simulink model "simTopLevel"  (R2016b)
settings: Solver=ode15s  StartTime=0.0  StopTime=2  RelTol=1e-3  EnableMultiTasking=on
InitFcn:
  | % minitaurParameters
model workspace (MAT data in the model file):
  MCOS : class17 (value not decoded)
  MCOS : class17 (value not decoded)
  MCOS : class17 (value not decoded)
  MCOS : class17 (value not decoded)
values from neighbouring files (symbols this model uses):
  controlParams = Simulink.Parameter(controlParams)    [minitaurParameters.m]
  envParams = Simulink.Parameter(envParams)    [minitaurParameters.m]
  IC = Simulink.Parameter(IC)    [minitaurParameters.m]
  minitaurParams = Simulink.Parameter(minitaurParams)    [minitaurParameters.m]
undefined symbols (not defined in the file or in its folder): Axis, Fn, ForeRearLag, Period, tau0, tau1, X, Y, Z
libraries: sm_lib x464, fl_lib x132, nesl_utility x41, Contact_Forces_Lib x28, simulink x13, simulink_extras x1
(part 13 of 13)

== system simTopLevel/GR Minitaur/minitaur_motor_module_IVB/DYS_BLDC_86x10_BE8108_12/DYS_BLDC_86x10_BE8108_12_stator_1_RIGID ==
  ReferenceFrame : sm_lib/Frames and Transforms/Reference Frame
  Solid : sm_lib/Body Elements/Solid  InertiaType=Custom  Mass=minitaurParams.Solid(6).mass  MassUnits=kg  CenterOfMass=minitaurParams.Solid(6).CoM  CenterOfMassUnits=mm  MomentsOfInertia=minitaurParams.Solid(6).MoI  MomentsOfInertiaUnits=kg*mm^2  ProductsOfInertia=minitaurParams.Solid(6).PoI  ProductsOfInertiaUnits=kg*mm^2  DensityBased=on  Density=1000  DensityUnits=kg/(m^3)  DoExposeReferenceFrame=on  SerializedFrames=<Frames/>  GraphicType=FromGeometry  MarkerShape=Sphere  MarkerSize=10  GraphicVisPropType=SimpleVisualProperties  GraphicDiffuseColor=minitaurParams.Solid(6).color  GraphicSpecularColor=[0.5 0.5 0.5 1.0]  GraphicAmbientColor=[0.15 0.15 0.15 1.0]  GraphicEmissiveColor=[0.0 0.0 0.0 1.0]  GraphicShininess=75  GraphicOpacity=minitaurParams.Solid(6).opacity  GeometryShape=FromFile  RectangleSize=[1 1]  RectangleSizeUnits=m  BrickDimensions=[1 1 1]  BrickDimensionUnits=m  CylinderRadius=1  CylinderRadiusUnits=m  CylinderLength=1  CylinderLengthUnits=m  SphereRadius=1  SphereRadiusUnits=m  EllipsoidRadii=[1 1 1]  EllipsoidRadiiUnits=m  ExtrusionCrossSection=[1 1; -1 1; -1 -1; 1 -1]  ExtrusionCrossSectionUnits=m  ExtrusionLength=1  ExtrusionLengthUnits=m  PolygonNumSides=3  PolygonOuterRadius=1  PolygonOuterRadiusUnits=m  ExtGeomFileType=STEP  ExtGeomFileName=model/DYS-BLDC-86x10-BE8108-12-stator_Default_sldprt.STEP  ExtGeomFileUnits=m  RevolutionCrossSection=[1 1; 1 -1; 2 -1; 2 1]  RevolutionCrossSectionUnits=m  RevolutionExtent=Full  RevolutionAngle=180  RevolutionAngleUnits=deg
  Transform : sm_lib/Frames and Transforms/Rigid Transform  TranslationMethod=Cartesian  TranslationStandardOffset=0  TranslationLengthUnit=mm  TranslationStandardAxis=+Z  TranslationCartesianOffset=minitaurParams.RigidTransform(17).translation  TranslationROffset=0  TranslationROffsetUnits=m  TranslationZOffset=0  TranslationZOffsetUnits=m  TranslationThetaOffset=0  TranslationThetaOffsetUnits=deg  RotationMethod=ArbitraryAxis  RotationAngleUnits=rad  RotationStandardAxis=+Z  RotationAngle=minitaurParams.RigidTransform(17).angle  RotationArbitraryAxis=minitaurParams.RigidTransform(17).axis  FollAlignAxisA=+X  BaseAlignAxisA=+Y  FollAlignAxisB=+Y  BaseAlignAxisB=+Z  RotationSequenceAxes=FollowerAxes  RotationSequence=XYX  RotationSequenceAngles=[0 0 0]  RotationSequenceAnglesUnits=deg  RotationMatrix=[1 0 0; 0 1 0; 0 0 1]
  Transform1 : sm_lib/Frames and Transforms/Rigid Transform  TranslationMethod=Cartesian  TranslationStandardOffset=0  TranslationLengthUnit=mm  TranslationStandardAxis=+Z  TranslationCartesianOffset=minitaurParams.RigidTransform(19).translation  TranslationROffset=0  TranslationROffsetUnits=m  TranslationZOffset=0  TranslationZOffsetUnits=m  TranslationThetaOffset=0  TranslationThetaOffsetUnits=deg  RotationMethod=ArbitraryAxis  RotationAngleUnits=rad  RotationStandardAxis=+Z  RotationAngle=minitaurParams.RigidTransform(19).angle  RotationArbitraryAxis=minitaurParams.RigidTransform(19).axis  FollAlignAxisA=+X  BaseAlignAxisA=+Y  FollAlignAxisB=+Y  BaseAlignAxisB=+Z  RotationSequenceAxes=FollowerAxes  RotationSequence=XYX  RotationSequenceAngles=[0 0 0]  RotationSequenceAnglesUnits=deg  RotationMatrix=[1 0 0; 0 1 0; 0 0 1]
  Transform2 : sm_lib/Frames and Transforms/Rigid Transform  TranslationMethod=Cartesian  TranslationStandardOffset=0  TranslationLengthUnit=mm  TranslationStandardAxis=+Z  TranslationCartesianOffset=minitaurParams.RigidTransform(26).translation  TranslationROffset=0  TranslationROffsetUnits=m  TranslationZOffset=0  TranslationZOffsetUnits=m  TranslationThetaOffset=0  TranslationThetaOffsetUnits=deg  RotationMethod=ArbitraryAxis  RotationAngleUnits=rad  RotationStandardAxis=+Z  RotationAngle=minitaurParams.RigidTransform(26).angle  RotationArbitraryAxis=minitaurParams.RigidTransform(26).axis  FollAlignAxisA=+X  BaseAlignAxisA=+Y  FollAlignAxisB=+Y  BaseAlignAxisB=+Z  RotationSequenceAxes=FollowerAxes  RotationSequence=XYX  RotationSequenceAngles=[0 0 0]  RotationSequenceAnglesUnits=deg  RotationMatrix=[1 0 0; 0 1 0; 0 0 1]
  Transform3 : sm_lib/Frames and Transforms/Rigid Transform  TranslationMethod=Cartesian  TranslationStandardOffset=0  TranslationLengthUnit=mm  TranslationStandardAxis=+Z  TranslationCartesianOffset=minitaurParams.RigidTransform(62).translation  TranslationROffset=0  TranslationROffsetUnits=m  TranslationZOffset=0  TranslationZOffsetUnits=m  TranslationThetaOffset=0  TranslationThetaOffsetUnits=deg  RotationMethod=ArbitraryAxis  RotationAngleUnits=rad  RotationStandardAxis=+Z  RotationAngle=minitaurParams.RigidTransform(62).angle  RotationArbitraryAxis=minitaurParams.RigidTransform(62).axis  FollAlignAxisA=+X  BaseAlignAxisA=+Y  FollAlignAxisB=+Y  BaseAlignAxisB=+Z  RotationSequenceAxes=FollowerAxes  RotationSequence=XYX  RotationSequenceAngles=[0 0 0]  RotationSequenceAnglesUnits=deg  RotationMatrix=[1 0 0; 0 1 0; 0 0 1]
  F2 : PMIOPort  Port=1  Side=Left
  F3 : PMIOPort  Port=2  Side=Left
  F : PMIOPort  Port=3  Side=Left
  F1 : PMIOPort  Port=4  Side=Right
  connections:
  ReferenceFrame/RConn1 -- Solid/RConn1 -- Transform/LConn1 -- Transform1/LConn1 -- Transform2/LConn1 -- Transform3/LConn1
  Transform/RConn1 -- F/RConn1
  Transform1/RConn1 -- F1/RConn1
  Transform2/RConn1 -- F2/RConn1
  Transform3/RConn1 -- F3/RConn1

== matlab function simTopLevel/Controller/Subsystem1/Minitaur Leg Actuator Coordinates to Configuration Coordinates1 ==
  data: p output; a input; l1 input; l2 input
function p = legIK(a, l1, l2)
% Converts between commanded (r,theta) to motor (thetaA,thetaB)
% a is (psi, r).
    psi=a(1)+pi/2;
    
    phi=acos((l1^2+a(2)^2-l2^2)/(2*l1*a(2)));
   
    p = zeros(2,1);
    p(1) = phi-psi-pi;
    p(2) = pi-(phi+psi);
    
end

== matlab function simTopLevel/Controller/Subsystem2/Minitaur Leg Actuator Coordinates to Configuration Coordinates1 ==
  data: p output; a input; l1 input; l2 input
function p = legIK(a, l1, l2)
% Converts between commanded (r,theta) to motor (thetaA,thetaB)
% a is (psi, r).
    psi=a(1)+pi/2;
    
    phi=acos((l1^2+a(2)^2-l2^2)/(2*l1*a(2)));
   
    p = zeros(2,1);
    p(1) = phi-psi-pi;
    p(2) = pi-(phi+psi);
    
end

== matlab function simTopLevel/Controller/Subsystem3/Minitaur Leg Actuator Coordinates to Configuration Coordinates1 ==
  data: p output; a input; l1 input; l2 input
function p = legIK(a, l1, l2)
% Converts between commanded (r,theta) to motor (thetaA,thetaB)
% a is (psi, r).
    psi=a(1)+pi/2;
    
    phi=acos((l1^2+a(2)^2-l2^2)/(2*l1*a(2)));
   
    p = zeros(2,1);
    p(1) = phi-psi-pi;
    p(2) = pi-(phi+psi);
    
end

== matlab function simTopLevel/Controller/Subsystem4/Minitaur Leg Actuator Coordinates to Configuration Coordinates1 ==
  data: p output; a input; l1 input; l2 input
function p = legIK(a, l1, l2)
% Converts between commanded (r,theta) to motor (thetaA,thetaB)
% a is (psi, r).
    psi=a(1)+pi/2;
    
    phi=acos((l1^2+a(2)^2-l2^2)/(2*l1*a(2)));
   
    p = zeros(2,1);
    p(1) = phi-psi-pi;
    p(2) = pi-(phi+psi);
    
end

== matlab function simTopLevel/Controller/Trajectory Planner/Elliptical Trajectory/Ellipse Trajectory ==
  data: r0 input; L1 output; L2 output; L3 output; L4 output; t input; ry input; rx input; thetaTilt input; theta1 output; theta2 output; theta3 output; theta4 output
function [ L1,L2,L3,L4,theta1,theta2,theta3,theta4] = EllipseTrajectory(r0,t,ry,rx,thetaTilt)
t=t*2*pi; % time in cycle
r1=[rx*cos(t(1)), -ry*sin(t(1))]';
r2=[rx*cos(t(2)), -ry*sin(t(2))]';
r3=[rx*cos(t(3)), -ry*sin(t(3))]';
r4=[rx*cos(t(4)), -ry*sin(t(4))]';

rot=[cos(thetaTilt) -sin(thetaTilt); sin(thetaTilt) cos(thetaTilt)];
r1=rot*r1+[0 r0]';
r2=rot*r2+[0 r0]';
r3=rot*r3+[0 r0]';
r4=rot*r4+[0 r0]';


L1=norm(r1);
L2=norm(r2);
L3=norm(r3); 
L4=norm(r4);
% theta1=acos(r1(1)/L1); 
% theta2=acos(r2(1)/L2); 
% theta3=acos(r3(1)/L3); 
% theta4=acos(r4(1)/L4);
% 
theta1=atan2(r1(2),r1(1));
theta2=atan2(r2(2),r2(1));
theta3=atan2(r3(2),r3(1));
theta4=atan2(r4(2),r4(1));
